simulink model "sim6TV2"  (R2019a)
settings: Solver=ode1  StartTime=0.0  StopTime=10  FixedStep=0.00001  RelTol=1e-3
values from neighbouring files (symbols this model uses):
  topology = [-2  1  0  0  0  1, ... (first row only)    [init6T.m]
  x0 = rand(8*6,1)+10    [init6T.m]
  xr0 = [1 0 1 0 1 0 1 0]    [init6T.m]
settings Model: Creator=zxz  LastModifiedBy=zxz

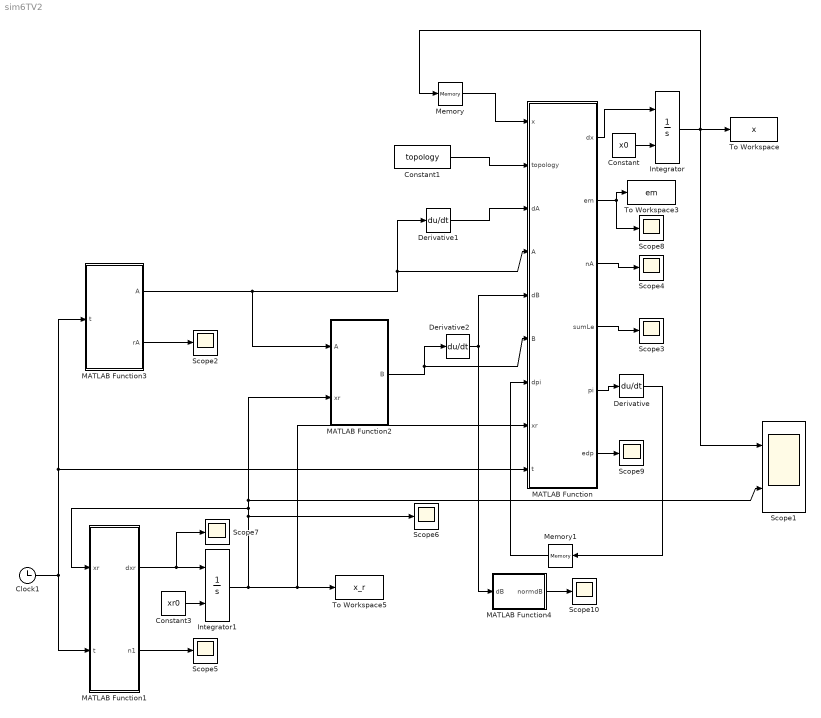
== system sim6TV2 ==
  Clock1 : Clock
  Constant : Constant  Value=x0
  Constant1 : Constant  Value=topology
  Constant3 : Constant  Value=xr0
  Derivative : Derivative
  Derivative1 : Derivative
  Derivative2 : Derivative
  Integrator : Integrator  InitialConditionSource=external
  Integrator1 : Integrator  InitialConditionSource=external
  MATLAB Function : MATLAB Function  TreatAsAtomicUnit=on
  MATLAB Function1 : MATLAB Function  TreatAsAtomicUnit=on
  MATLAB Function2 : MATLAB Function  TreatAsAtomicUnit=on
  MATLAB Function3 : MATLAB Function  TreatAsAtomicUnit=on
  MATLAB Function4 : MATLAB Function  TreatAsAtomicUnit=on
  Memory : Memory
  Memory1 : Memory
  Scope1 : Scope  NumInputPorts=2
  Scope{2..10} (9 alike) : Scope
  To Workspace : ToWorkspace  VariableName=x  SampleTime=-1
  To Workspace3 : ToWorkspace  VariableName=em  SampleTime=-1
  To Workspace5 : ToWorkspace  VariableName=x_r  SampleTime=-1
  wires:
  MATLAB Function/1(dx) -> Integrator/1
  Integrator/1 -> Scope1/1, Memory/1, To Workspace/1
  Constant/1 -> Integrator/2
  Constant1/1 -> MATLAB Function/2(topology)
  Clock1/1 -> MATLAB Function/9(t), MATLAB Function3/1(t), MATLAB Function1/2(t)
  MATLAB Function/2(em) -> Scope8/1, To Workspace3/1
  MATLAB Function2/1(B) -> Derivative2/1, MATLAB Function/6(B)
  MATLAB Function3/1(A) -> MATLAB Function2/1(A), Derivative1/1, MATLAB Function/4(A)
  Derivative1/1 -> MATLAB Function/3(dA)
  Memory/1 -> MATLAB Function/1(x)
  MATLAB Function/3(nA) -> Scope4/1
  MATLAB Function/4(sumLe) -> Scope3/1
  MATLAB Function1/1(dxr) -> Scope7/1, Integrator1/1
  Integrator1/1 -> To Workspace5/1, MATLAB Function/8(xr), MATLAB Function1/1(xr), MATLAB Function2/2(xr), Scope1/2, Scope6/1
  Constant3/1 -> Integrator1/2
  Derivative2/1 -> MATLAB Function/5(dB), MATLAB Function4/1(dB)
  MATLAB Function3/2(rA) -> Scope2/1
  MATLAB Function1/2(n1) -> Scope5/1
  MATLAB Function/6(edp) -> Scope9/1
  MATLAB Function/5(pi) -> Derivative/1
  Derivative/1 -> Memory1/1
  Memory1/1 -> MATLAB Function/7(dpi)
  MATLAB Function4/1(normdB) -> Scope10/1

== matlab function sim6TV2/MATLAB Function1 ==
  data: xr input; t input; dxr output; n1 output
function [dxr,n1]= fcn(xr,t)

Ae=[ 0  1  0  1  0  1  0  1,
    -1  0  1 -1  0  0  0  0,
     0 -1  0  0  0  0  1  1,
    -1  1  0  0  0  0  0  0,
     0  0  0  0  0  0  0  0,
    -1  0  0  0  0  0  1  2,
     0  0 -1  0  0 -1  0  0,
    -1  0 -1  0  0 -2  0  0];


dxr=Ae*xr;

n1=sum(abs(dxr));

== matlab function sim6TV2/MATLAB Function ==
  data: x input; dx output; topology input; dA input; A input; dB input; B input; em output; nA output; sumLe output; dpi input; pi output; edp output; xr input; t input
function [dx,em,nA,sumLe,pi,edp] = fcn(x,topology,dA,A,dB,B,dpi,xr,t)

dx=zeros(48,1);
alpha=14;
k0=5;
k2=10;
em=zeros(6,1);
nA=zeros(6,1);
sumLe=zeros(48,1);
pi=zeros(8,8);
II8=[1 1 1 1 1 1 1 1];
for i=1:6
    Ai=1;
    Bi=1;
    dAi=1;
    dBi=1;
    if(i==1)
        Ai  = A(1:2,:);
        dAi = dA(1:2,:);
        Bi  = B(1:2,:);
        dBi = dB(1:2,:);
    end
    if(i==2)
        Ai  = A(3,:);
        dAi = dA(3,:);
        Bi  = B(3,:);
        dBi = dB(3,:);
    end
    if(i==3)
        Ai  = A(4:5,:);
        dAi = dA(4:5,:);
        Bi  = B(4:5,:);
        dBi = dB(4:5,:);
    end
    if(i==4)
        Ai  = A(6,:);
        dAi = dA(6,:);
        Bi  = B(6,:);
        dBi = dB(6,:);
    end
    if(i==5)
        Ai  = A(7,:);
        dAi = dA(7,:);
        Bi  = B(7,:);
        dBi = dB(7,:);
    end
    if(i==6)
        Ai  = A(8,:);
        dAi = dA(8,:);
        Bi  = B(8,:);
        dBi = dB(8,:);
    end
    pi=diag(ones(1,8))-Ai'*(Ai*Ai')^(-1)*Ai;
    
    dx(8*(i-1)+1:8*(i-1)+8) = -k0*Ai'*(Ai*Ai')^(-1)*(Ai*x(8*(i-1)+1:8*(i-1)+8)-Bi);
    dx(8*(i-1)+1:8*(i-1)+8) = dx(8*(i-1)+1:8*(i-1)+8)-Ai'*(Ai*Ai')^(-1)*(dAi*x(8*(i-1)+1:8*(i-1)+8)-dBi);
%     dx(8*(i-1)+1:8*(i-1)+8) = dx(8*(i-1)+1:8*(i-1)+8)  -alpha*Ai'*(Ai*Ai')^(-1)*sign(Ai*x(8*(i-1)+1:8*(i-1)+8)-Bi);
    dx(8*(i-1)+1:8*(i-1)+8) = dx(8*(i-1)+1:8*(i-1)+8)-Ai'*(Ai*Ai')^(-1)*dAi*x(8*(i-1)+1:8*(i-1)+8);
    em(i)=norm(Ai*x(8*(i-1)+1:8*(i-1)+8)-Bi);
    
    tmp=zeros(8,1);

    for j=1:6
        if(topology(i,j)<0.5||i==j) continue;
        end
        %dx(8*(i-1)+1:8*(i-1)+8) = dx(8*(i-1)+1:8*(i-1)+8)- k2*pi*sign(pi*(x(8*(i-1)+1:8*(i-1)+8)-x(8*(j-1)+1:8*(j-1)+8)));
        tmp=tmp + (x(8*(i-1)+1:8*(i-1)+8)-x(8*(j-1)+1:8*(j-1)+8));
        sumLe(8*(i-1)+1:8*(i-1)+8) =sumLe(8*(i-1)+1:8*(i-1)+8) +abs(x(8*(i-1)+1:8*(i-1)+8)-x(8*(j-1)+1:8*(j-1)+8));
    end
    nA(i)=norm(dAi/norm(Ai));


    dx(8*(i-1)+1:8*(i-1)+8) = dx(8*(i-1)+1:8*(i-1)+8)- k2*pi*sign(pi*tmp);
%     dx(8*(i-1)+1:8*(i-1)+8) = dx(8*(i-1)+1:8*(i-1)+8)- k2*pi*(tmp);
end
pi=diag(ones(1,8))-Ai'*(Ai*Ai')^(-1)*Ai;
% test=-dAi'*(Ai*Ai')^(-1)*Ai - Ai'*(Ai*Ai')^(-1)*dAi + Ai'*(Ai*Ai')^(-2)*(dAi*Ai'+Ai*dAi')*Ai;
test=-dAi'*(Ai*Ai')^(-1)*Ai - Ai'*(Ai*Ai')^(-1)*dAi + 2*Ai'*(Ai*Ai')^(-2)*dAi*Ai'*Ai;
% if(norm(dAi)>1)
%     aa=1;
% end
edp=norm(test-dpi);
% edp=norm(dAi'*((Ai*Ai')^(-1))*Ai-Ai'*((Ai*Ai')^(-1))*dAi);
end

== matlab function sim6TV2/MATLAB Function2 ==
  data: A input; B output; xr input
function B = fcn(A,xr)

B=A*xr;

== matlab function sim6TV2/MATLAB Function3 ==
  data: t input; A output; rA output
function [A, rA] = fcn(t)

% A=[ 1            1 1 1 1 1 1 1,
%     2+cos(0.7*t) 1 1 1 1 1 1 0,
%     2+cos(0.6*t) 1 1 1 1 1 0 0,
%     2+cos(0.5*t) 1 1 1 1 0 0 0,
%     2+sin(0.4*t) 1 1 1 0 0 0 0,
%     2+sin(0.4*t) 1 1 0 0 0 0 0,
%     2+sin(0.4*t) 1 0 0 0 0 0 0,
%     2+sin(0.4*t) 0 0 0 0 0 0 1];
A=[ 1            1 1 1 1 1 1 0,
    2+cos(0.7*t) 1 1 1 1 1 0 1,
    2+cos(0.6*t) 1 1 1 1 1 1 0,
    2+cos(0.5*t) 1 1 1 1 0 0 1,
    2+sin(0.4*t) 1 1 1 0 0 1 0,
    2+sin(0.4*t) 1 1 0 0 0 0 1,
    2+sin(0.4*t) 1 0 0 0 0 1 0,
    2+sin(0.4*t) 0 0 0 0 0 0 1];
% A=[ 1            1 1 1 1 1 1 1,
%     2+cos(7*t) 1 1 1 1 1 1 0,
%     2+cos(6*t) 1 1 1 1 1 0 0,
%     2+cos(5*t) 1 1 1 1 0 0 0,
%     2+sin(4*t) 1 1 1 0 0 0 0,
%     2+sin(3*t) 1 1 0 0 0 0 0,
%     2+sin(2*t) 1 0 0 0 0 0 0,
%     2+sin(1*t) 0 0 0 0 0 0 1];
% A=[ 1            1 1 1 1 1 1 1,
%     2 1 1 1 1 1 1 0,
%     2 1 1 1 1 1 0 0,
%     2 1 1 1 1 0 0 0,
%     2 1 1 1 0 0 0 0,
%     2 1 1 0 0 0 0 0,
%     2 1 0 0 0 0 0 0,
%     2 0 0 0 0 0 0 1];

rA=rank(A);

== matlab function sim6TV2/MATLAB Function4 ==
  data: dB input; normdB output
function normdB  = fcn(dB)
normdB=norm(dB);
